simulink model "Q7_3"  (R2020b)
settings: Solver=VariableStepAuto  StartTime=0.0  StopTime=10.0  RelTol=1e-3
settings Model: Creator=Javad  LastModifiedBy=Javad

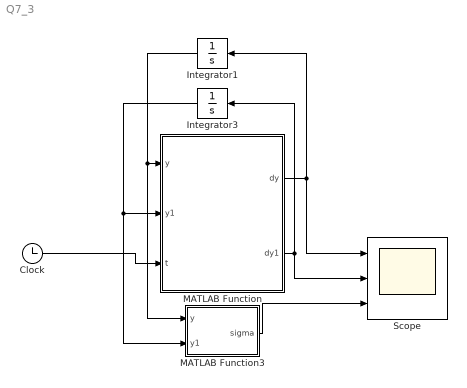
== system Q7_3 ==
  Clock : Clock
  Integrator1 : Integrator  InitialCondition=1
  Integrator3 : Integrator  InitialCondition=1
  MATLAB Function : MATLAB Function  TreatAsAtomicUnit=on
  MATLAB Function3 : MATLAB Function  TreatAsAtomicUnit=on
  Scope : Scope  NumInputPorts=3
  wires:
  Clock/1 -> MATLAB Function/3(t)
  MATLAB Function/1(dy) -> Integrator1/1, Scope/1
  Integrator1/1 -> MATLAB Function3/1(y), MATLAB Function/1(y)
  MATLAB Function/2(dy1) -> Integrator3/1, Scope/2
  Integrator3/1 -> MATLAB Function3/2(y1), MATLAB Function/2(y1)
  MATLAB Function3/1(sigma) -> Scope/3

== matlab function Q7_3/MATLAB Function ==
  data: y input; y1 input; dy output; t input; dy1 output
function [dy,dy1] = sys(y,y1,t)
b1=1;
b2=2;
b3=3;
k1=4;
k3=5;
mt=1/(t+1);
c=0.5;
if y>0.9
    dy1=0;
end
u=(b1+b2*abs(y1))+b3*sign(y1)+(k1+k3*y^2)+sin(pi*t)+c*mt*dy1;
dy=y1;
dy1=(1/mt)*(- (b1+b2*abs(y1)) - b3*sign(y1)- (k1+k3*y^2)*y+ u - sin(pi*t));

== matlab function Q7_3/MATLAB Function3 ==
  data: y input; sigma output; y1 input
function sigma = surface1(y,y1)
sigma=y1+0.5*y;
